simulink model "motor_passo"  (R2022b)
settings: Solver=ode45  StartTime=0.0  StopTime=0.2  RelTol=1e-3  EnableMultiTasking=on
values from neighbouring files (symbols this model uses):
  B = 1e-3    (= 0.001)    [loop_sim.m]    (also in sim_motor.m = Bs(i); var_passo.m)
  J = 2e-5    (= 2e-05)    [loop_sim.m]    (also in var_passo.m)
  Ls = 1e-3    (= 0.001)    [loop_sim.m]    (also in sim_motor.m = LSs(i); var_passo.m)
  p = 360 / (2*m*stepsize)    (= 3)    [loop_sim.m]    (also in var_passo.m)
  psim = 0.04    [loop_sim.m]    (also in sim_motor.m = PSIs(i); var_passo.m)
  Rs = 1.2    [loop_sim.m]    (also in sim_motor.m = RSs(i); var_passo.m)
  theta0 = 0    [loop_sim.m]    (also in var_passo.m)
  TL = 0.2    [loop_sim.m]    (also in var_passo.m)
libraries: spsControlledCurrentSourceLib x2, spsControlledVoltageSourceLib x2, spsParallelRLCBranchLib x2, spsVoltageMeasurementLib x2, sps_lib x1
settings Model: Creator=11802972  LastModifiedBy=andre
settings SolverCC: AlgebraicLoopSolver=TrustRegion
settings DataIOCC: LimitDataPoints=on  SaveFormat=Array  ReturnWorkspaceOutputs=off
settings OptimizationCC: LifeSpan=inf
settings DebuggingCC: UnconnectedInputMsg=warning  UnconnectedOutputMsg=warning  UnconnectedLineMsg=warning  SFUnexpectedBacktrackingDiag=warning  SFNoUnconditionalDefaultTransitionDiag=warning  SFExecutionAtInitializationDiag=none  SFMachineParentedDataDiag=warning  ArithmeticOperatorsInVariantConditions=warning
settings HardwareCC: ProdBitPerPointer=32  ProdBitPerSizeT=32  ProdBitPerPtrDiffT=32  ProdLargestAtomicFloat=None  ProdIntDivRoundTo=Undefined  ProdEndianess=Unspecified  ProdWordSize=32  ProdHWDeviceType=32-bit Generic
settings ModelReferenceCC: PropagateSignalLabelsOutOfModel=off
settings SFSimCC: SimUseLocalCustomCode=off  CustomCodeUndefinedFunction=UseInterfaceOnly
settings RTWCC: RTWUseLocalCustomCode=off
settings CodeAppCC: StateflowObjectComments=on
settings GRTTargetCC: TargetLangStandard=C89/C90 (ANSI)
settings ConfigComp: CovMetricSettings=dw  CovSaveCumulativeToWorkspaceVar=on  CovSaveSingleToWorkspaceVar=on  CovExternalEMLEnable=off
settings SimscapeCC: SimscapeNormalizeSystem=off

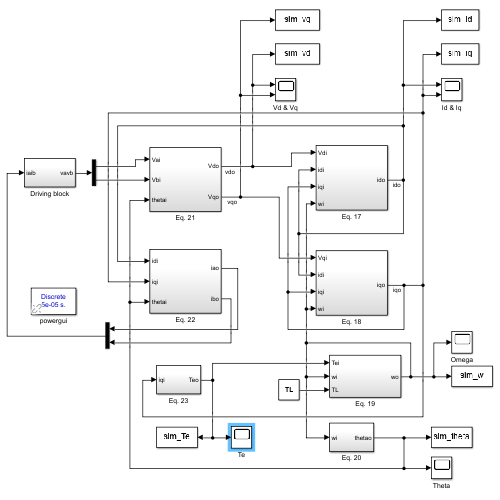
[thumbnail: Simulink's stored preview of the top-level diagram]
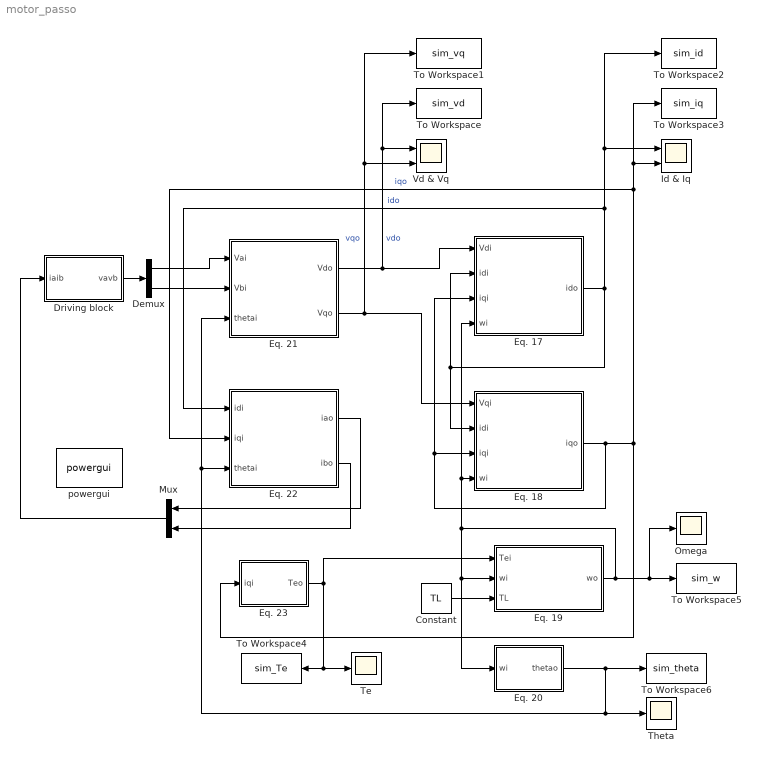
== system motor_passo ==
  Constant : Constant  Value=TL
  Demux : Demux  Outputs=2
  Driving block : Subsystem
  Eq. 17 : Subsystem
  Eq. 18 : Subsystem
  Eq. 19 : Subsystem
  Eq. 20 : Subsystem
  Eq. 21 : Subsystem
  Eq. 22 : Subsystem
  Eq. 23 : Subsystem
  Id & Iq : Scope  NumInputPorts=2
  Mux : Mux  Inputs=2
  Omega : Scope
  Te : Scope
  Theta : Scope
  To Workspace : ToWorkspace  VariableName=sim_vd  SaveFormat=Timeseries  SampleTime=-1
  To Workspace1 : ToWorkspace  VariableName=sim_vq  SaveFormat=Timeseries  SampleTime=-1
  To Workspace2 : ToWorkspace  VariableName=sim_id  SaveFormat=Timeseries  SampleTime=-1
  To Workspace3 : ToWorkspace  VariableName=sim_iq  SaveFormat=Timeseries  SampleTime=-1
  To Workspace4 : ToWorkspace  VariableName=sim_Te  SaveFormat=Timeseries  SampleTime=-1
  To Workspace5 : ToWorkspace  VariableName=sim_w  SaveFormat=Timeseries  SampleTime=-1
  To Workspace6 : ToWorkspace  VariableName=sim_theta  SaveFormat=Timeseries  SampleTime=-1
  Vd & Vq : Scope  NumInputPorts=2
  powergui : sps_lib/powergui  Priority=1  SimulationMode=Discrete  SampleTime=50e-6  frequency=60  Iterations=50  frequencyindice=0  Pbase=100e6  ErrMax=1e-4  UnitsV=kV  UnitsW=MW  buscounter=0  FunctionMessages=off  echomessages=off  EnableUseOfTLC=off  CurrentSourceSwitches=off  DisableSnubberDevices=off  DisableRonSwitches=off  DisableVfSwitches=off  DisplayEquations=off  AutomaticDiscreteSolvers=off  SolverType=Tustin/Backward Euler (TBE)  Interpol=off  ExternalGateDelay=off  methode=off  Ts=100  x0status=blocks  SPID=off  SwTol=0  HookPort=off  NonlinearTolerance=1e-4  nMaxIteration=100  ContinueOnMaxIteration=off  RestoreLinks=warning  ResistiveCurrentMeasurement=off  Frange=[0:2:500]  Ylog=off  Xlog=on  ShowGrid=off  save=off  variable=ZData  structure=0  ZoomFFT=off  StartTime=0.0  cycles=1  DisplayStyle=1  fundamental=60  FreqAxis=off  MaxFrequency=1000  frequencyindicesteady=1  RmsSteady=1  display=off
  wires:
  Eq. 21/1(Vdo) -> Eq. 17/1(Vdi), To Workspace/1, Vd & Vq/1  "vdo"
  Eq. 21/2(Vqo) -> Eq. 18/1(Vqi), To Workspace1/1, Vd & Vq/2  "vqo"
  Eq. 23/1(Teo) -> Te/1, To Workspace4/1, Eq. 19/1(Tei)
  Driving block/1(vavb) -> Demux/1
  Constant/1 -> Eq. 19/3(TL)
  Eq. 17/1(ido) -> To Workspace2/1, Id & Iq/1, Eq. 22/1(idi), Eq. 17/2(idi), Eq. 18/2(idi)  "ido"
  Eq. 18/1(iqo) -> Eq. 18/3(iqi), Eq. 17/3(iqi), Eq. 23/1(iqi), To Workspace3/1, Id & Iq/2, Eq. 22/2(iqi)  "iqo"
  Eq. 19/1(wo) -> Omega/1, To Workspace5/1, Eq. 17/4(wi), Eq. 18/4(wi), Eq. 20/1(wi), Eq. 19/2(wi)
  Eq. 22/1(iao) -> Mux/1
  Eq. 22/2(ibo) -> Mux/2
  Mux/1 -> Driving block/1(iaib)
  Demux/1 -> Eq. 21/1(Vai)
  Demux/2 -> Eq. 21/2(Vbi)
  Eq. 20/1(thetao) -> To Workspace6/1, Theta/1, Eq. 22/3(thetai), Eq. 21/3(thetai)

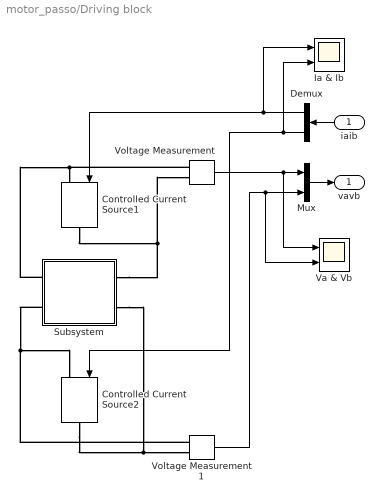
== system motor_passo/Driving block ==
  iaib : Inport
  Controlled Current Source1 : spsControlledCurrentSourceLib/Controlled Current Source  Initialize=on  Source_Type=AC  Amplitude=0  Phase=0  Frequency=0  Measurements=None
  Controlled Current Source2 : spsControlledCurrentSourceLib/Controlled Current Source  Initialize=on  Source_Type=AC  Amplitude=0  Phase=0  Frequency=0  Measurements=None
  Demux : Demux  Outputs=2
  Ia & Ib : Scope  NumInputPorts=2
  Mux : Mux  Inputs=2
  Subsystem : Subsystem
  Va & Vb : Scope  NumInputPorts=2
  Voltage Measurement : spsVoltageMeasurementLib/Voltage Measurement  PhasorSimulation=off  OutputType=Complex  PSBequivalent=0
  Voltage Measurement1 : spsVoltageMeasurementLib/Voltage Measurement  PhasorSimulation=off  OutputType=Complex  PSBequivalent=0
  vavb : Outport
  wires:
  iaib/1 -> Demux/1
  Mux/1 -> vavb/1
  Voltage Measurement/1 -> Va & Vb/1, Mux/1
  Demux/1 -> Ia & Ib/1, Controlled Current Source1/1
  Demux/2 -> Ia & Ib/2, Controlled Current Source2/1
  Voltage Measurement1/1 -> Va & Vb/2, Mux/2
  connections:
  Subsystem/RConn1 -- Controlled Current Source1/RConn1 -- Voltage Measurement/LConn2
  Voltage Measurement/LConn1 -- Subsystem/LConn1 -- Controlled Current Source1/LConn1
  Subsystem/LConn2 -- Voltage Measurement1/LConn1 -- Controlled Current Source2/LConn1
  Subsystem/RConn2 -- Controlled Current Source2/RConn1 -- Voltage Measurement1/LConn2

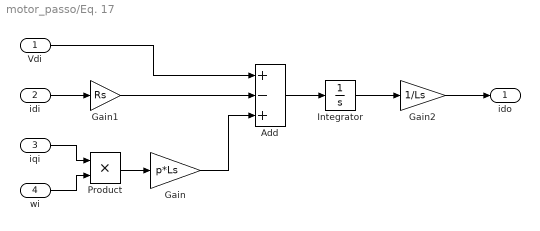
== system motor_passo/Eq. 17 ==
  Vdi : Inport
  idi : Inport  Port=2
  iqi : Inport  Port=3
  wi : Inport  Port=4
  Add : Sum  Inputs=+-+
  Gain : Gain  Gain=p*Ls
  Gain1 : Gain  Gain=Rs
  Gain2 : Gain  Gain=1/Ls
  Integrator : Integrator
  Product : Product
  ido : Outport
  wires:
  iqi/1 -> Product/1
  wi/1 -> Product/2
  Product/1 -> Gain/1
  idi/1 -> Gain1/1
  Vdi/1 -> Add/1
  Gain1/1 -> Add/2
  Gain/1 -> Add/3
  Add/1 -> Integrator/1
  Integrator/1 -> Gain2/1
  Gain2/1 -> ido/1

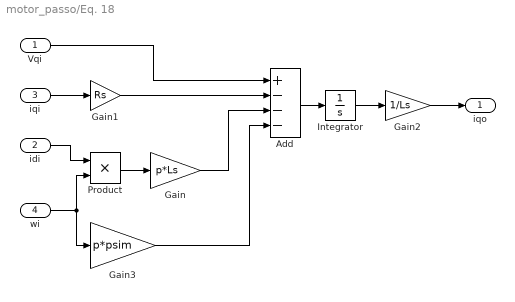
== system motor_passo/Eq. 18 ==
  Vqi : Inport
  idi : Inport  Port=2
  iqi : Inport  Port=3
  wi : Inport  Port=4
  Add : Sum  Inputs=+---
  Gain : Gain  Gain=p*Ls
  Gain1 : Gain  Gain=Rs
  Gain2 : Gain  Gain=1/Ls
  Gain3 : Gain  Gain=p*psim
  Integrator : Integrator
  Product : Product
  iqo : Outport
  wires:
  wi/1 -> Product/2, Gain3/1
  Product/1 -> Gain/1
  Vqi/1 -> Add/1
  Gain1/1 -> Add/2
  Gain/1 -> Add/3
  Add/1 -> Integrator/1
  Integrator/1 -> Gain2/1
  Gain2/1 -> iqo/1
  iqi/1 -> Gain1/1
  idi/1 -> Product/1
  Gain3/1 -> Add/4

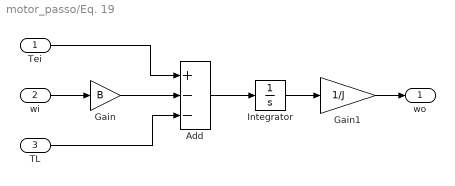
== system motor_passo/Eq. 19 ==
  Tei : Inport
  wi : Inport  Port=2
  TL : Inport  Port=3
  Add : Sum  Inputs=+--
  Gain : Gain  Gain=B
  Gain1 : Gain  Gain=1/J
  Integrator : Integrator
  wo : Outport
  wires:
  wi/1 -> Gain/1
  Tei/1 -> Add/1
  Gain/1 -> Add/2
  TL/1 -> Add/3
  Add/1 -> Integrator/1
  Integrator/1 -> Gain1/1
  Gain1/1 -> wo/1

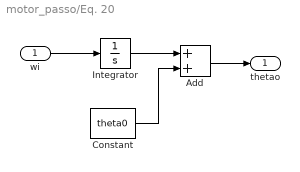
== system motor_passo/Eq. 20 ==
  wi : Inport
  Add : Sum
  Constant : Constant  Value=theta0
  Integrator : Integrator
  thetao : Outport
  wires:
  wi/1 -> Integrator/1
  Integrator/1 -> Add/1
  Constant/1 -> Add/2
  Add/1 -> thetao/1

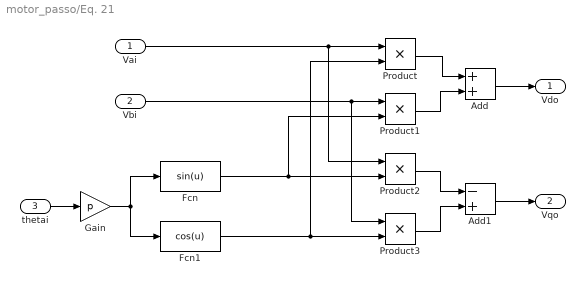
== system motor_passo/Eq. 21 ==
  Vai : Inport
  Vbi : Inport  Port=2
  thetai : Inport  Port=3
  Add : Sum
  Add1 : Sum  Inputs=-+
  Fcn : Fcn  Expr=sin(u)
  Fcn1 : Fcn  Expr=cos(u)
  Gain : Gain  Gain=p
  Product{,1..3} (4 alike) : Product
  Vdo : Outport
  Vqo : Outport  Port=2
  wires:
  thetai/1 -> Gain/1
  Gain/1 -> Fcn1/1, Fcn/1
  Product/1 -> Add/1
  Product1/1 -> Add/2
  Product2/1 -> Add1/1
  Product3/1 -> Add1/2
  Add1/1 -> Vqo/1
  Add/1 -> Vdo/1
  Vai/1 -> Product2/1, Product/1
  Vbi/1 -> Product3/1, Product1/1
  Fcn1/1 -> Product/2, Product3/2
  Fcn/1 -> Product1/2, Product2/2

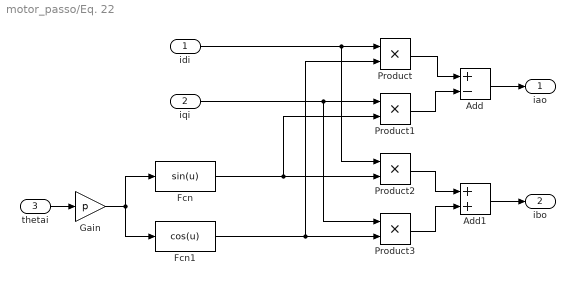
== system motor_passo/Eq. 22 ==
  idi : Inport
  iqi : Inport  Port=2
  thetai : Inport  Port=3
  Add : Sum  Inputs=+-
  Add1 : Sum
  Fcn : Fcn  Expr=sin(u)
  Fcn1 : Fcn  Expr=cos(u)
  Gain : Gain  Gain=p
  Product{,1..3} (4 alike) : Product
  iao : Outport
  ibo : Outport  Port=2
  wires:
  Gain/1 -> Fcn1/1, Fcn/1
  Product/1 -> Add/1
  Product1/1 -> Add/2
  Product2/1 -> Add1/1
  Product3/1 -> Add1/2
  Add1/1 -> ibo/1
  Add/1 -> iao/1
  Fcn1/1 -> Product/2, Product3/2
  Fcn/1 -> Product1/2, Product2/2
  thetai/1 -> Gain/1
  idi/1 -> Product2/1, Product/1
  iqi/1 -> Product3/1, Product1/1

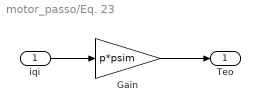
== system motor_passo/Eq. 23 ==
  iqi : Inport
  Gain : Gain  Gain=p*psim
  Teo : Outport
  wires:
  iqi/1 -> Gain/1
  Gain/1 -> Teo/1

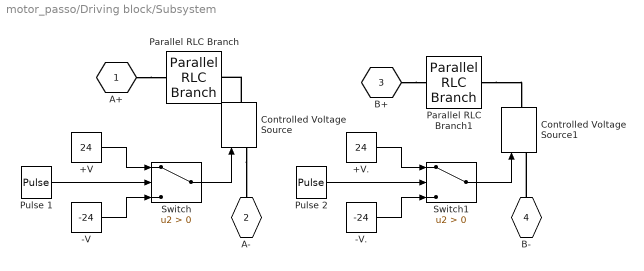
== system motor_passo/Driving block/Subsystem ==
  +V : Constant  Value=24
  +V. : Constant  Value=24
  -V : Constant  Value=-24
  -V. : Constant  Value=-24
  Controlled Voltage Source : spsControlledVoltageSourceLib/Controlled Voltage Source  Initialize=on  Source_Type=AC  Amplitude=0  Phase=0  Frequency=0  Measurements=None
  Controlled Voltage Source1 : spsControlledVoltageSourceLib/Controlled Voltage Source  Initialize=on  Source_Type=AC  Amplitude=0  Phase=0  Frequency=0  Measurements=None
  Parallel RLC Branch : spsParallelRLCBranchLib/Parallel RLC Branch  LConnTagsString=a  RConnTagsString=__new0  BranchType=R  Resistance=Rs  Inductance=1e-3  SetiL0=off  InitialCurrent=0  Capacitance=1e-6  Setx0=off  InitialVoltage=0  Measurements=None
  Parallel RLC Branch1 : spsParallelRLCBranchLib/Parallel RLC Branch  LConnTagsString=a  RConnTagsString=__new0  BranchType=R  Resistance=Rs  Inductance=1e-3  SetiL0=off  InitialCurrent=0  Capacitance=1e-6  Setx0=off  InitialVoltage=0  Measurements=None
  Pulse 1 : DiscretePulseGenerator  PulseType=Time based  Period=0.1  PulseWidth=50
  Pulse 2 : DiscretePulseGenerator  PulseType=Time based  Period=0.1  PulseWidth=50  PhaseDelay=0.025
  Switch : Switch  Criteria=u2 > Threshold  SaturateOnIntegerOverflow=off  InputSameDT=off
  Switch1 : Switch  Criteria=u2 > Threshold  SaturateOnIntegerOverflow=off  InputSameDT=off
  A+ : PMIOPort  Side=Left
  A- : PMIOPort  Port=2  Side=Right
  B+ : PMIOPort  Port=3  Side=Left
  B- : PMIOPort  Port=4  Side=Right
  wires:
  +V/1 -> Switch/1
  -V/1 -> Switch/3
  Pulse 1/1 -> Switch/2
  +V./1 -> Switch1/1
  -V./1 -> Switch1/3
  Pulse 2/1 -> Switch1/2
  Switch/1 -> Controlled Voltage Source/1
  Switch1/1 -> Controlled Voltage Source1/1
  connections:
  Controlled Voltage Source/LConn1 -- A-/RConn1
  B-/RConn1 -- Controlled Voltage Source1/LConn1
  A+/RConn1 -- Parallel RLC Branch/LConn1
  Controlled Voltage Source/RConn1 -- Parallel RLC Branch/RConn1
  Parallel RLC Branch1/RConn1 -- Controlled Voltage Source1/RConn1
  B+/RConn1 -- Parallel RLC Branch1/LConn1
